simulink model "simulationInAccurateModel"  (R2022b)
settings: Solver=VariableStepAuto  StartTime=0.0  StopTime=20.0  MaxStep=2e-3  RelTol=1e-3
values from neighbouring files (symbols this model uses):
  K_c_PI1 = 0.15/k+(0.35-(theta*tau)/(theta+tau)^2)*(tau/(k*theta))    (= 1899030.33908)    [simulation.m]
  K_c_PI2 = 1/k*(tau/(tau/3+theta))    (= 2117647.05882)    [simulation.m]
  K_c_PID1 = 1/k*(0.2+0.45*(tau/theta))    (= 3440000)    [simulation.m]
  K_c_PID2 = 1/k*(2*tau+theta)/(2*tau/3+theta)    (= 2655172.41379)    [simulation.m]
  tau_d_PID1 = (0.5*theta*tau)/(0.3*theta+tau)    (= 0.12)    [simulation.m]
  tau_d_PID2 = (tau*theta)/(2*tau+theta)    (= 0.116883116883)    [simulation.m]
  tau_i_PI1 = 0.35*theta+(13*theta*tau^2)/(tau^2+12*theta*tau+7*theta^2)    (= 1.24751101625)    [simulation.m]
  tau_i_PI2 = tau    (= 1.8)    [simulation.m]
  tau_i_PID1 = theta*(0.4*theta+0.8*tau)/(theta+0.1*tau)    (= 0.895348837209)    [simulation.m]
  tau_i_PID2 = tau+theta/2    (= 1.925)    [simulation.m]
undefined symbols (not defined in the file or in its folder): k_over, k_under, tau_over, tau_under, theta_over, theta_under
settings Model: Creator=omare  LastModifiedBy=omare
settings DataIOCC: ReturnWorkspaceOutputs=off

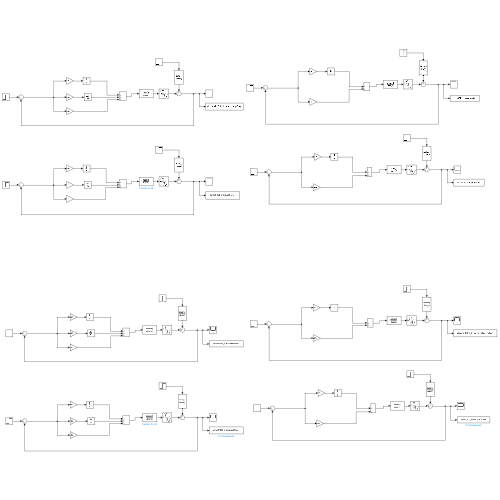
[thumbnail: Simulink's stored preview of the top-level diagram]
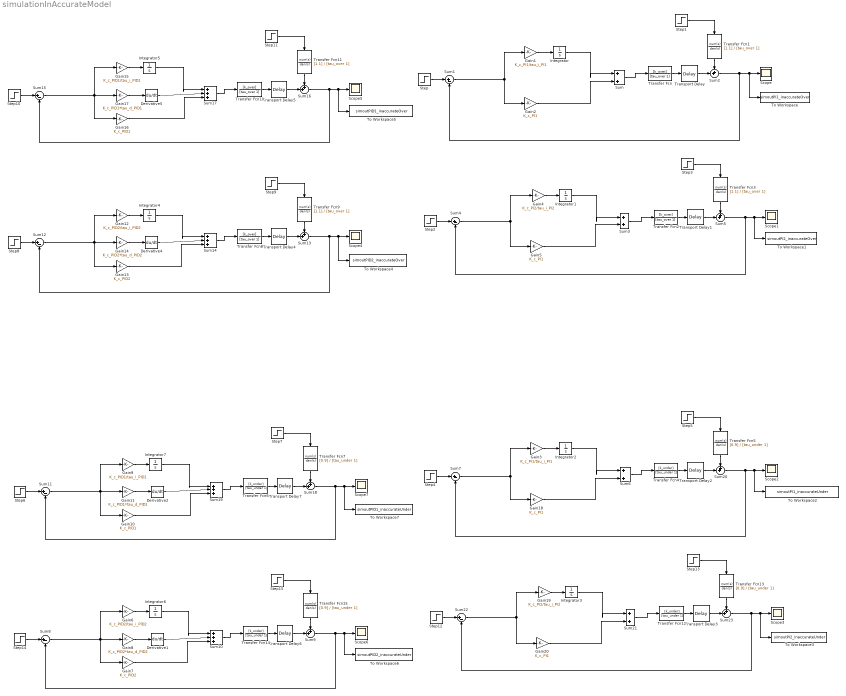
== system simulationInAccurateModel ==
  Derivative{1..2,4..5} (4 alike) : Derivative
  Gain1 : Gain  Gain=K_c_PI1/tau_i_PI1
  Gain10 : Gain  Gain=K_c_PID1
  Gain11 : Gain  Gain=K_c_PID1*tau_d_PID1
  Gain12 : Gain  Gain=K_c_PID2/tau_i_PID2
  Gain13 : Gain  Gain=K_c_PID2
  Gain14 : Gain  Gain=K_c_PID2*tau_d_PID2
  Gain15 : Gain  Gain=K_c_PID1/tau_i_PID1
  Gain16 : Gain  Gain=K_c_PID1
  Gain17 : Gain  Gain=K_c_PID1*tau_d_PID1
  Gain{2,5,18,20} (4 alike) : Gain  Gain=K_c_PI1
  Gain19 : Gain  Gain=K_c_PI2/tau_i_PI2
  Gain3 : Gain  Gain=K_c_PI1/tau_i_PI1
  Gain4 : Gain  Gain=K_c_PI2/tau_i_PI2
  Gain6 : Gain  Gain=K_c_PID2/tau_i_PID2
  Gain7 : Gain  Gain=K_c_PID2
  Gain8 : Gain  Gain=K_c_PID2*tau_d_PID2
  Gain9 : Gain  Gain=K_c_PID1/tau_i_PID1
  Integrator{,1..7} (8 alike) : Integrator
  Scope{,1..7} (8 alike) : Scope
  Step{,2,4,6,8,10,12,14} (8 alike) : Step  Time=0  SampleTime=0
  Step{1,3,5,7,9,11,13,15} (8 alike) : Step  Time=12  SampleTime=0
  Sum{,3,6,21} (4 alike) : Sum  Inputs=|++
  Sum{1,4,7..8,11..12,15,22} (8 alike) : Sum  Inputs=|+-
  Sum{10,14,17,19} (4 alike) : Sum  Inputs=|+++
  Sum{2,5,9,13,16,18,20,23} (8 alike) : Sum  Inputs=++|
  To Workspace : ToWorkspace  VariableName=simoutPI1_inaccurateOver  SaveFormat=Timeseries  SampleTime=-1
  To Workspace1 : ToWorkspace  VariableName=simoutPI2_inaccurateOver  SaveFormat=Timeseries  SampleTime=-1
  To Workspace2 : ToWorkspace  VariableName=simoutPI1_inaccurateUnder  SaveFormat=Timeseries  SampleTime=-1
  To Workspace3 : ToWorkspace  VariableName=simoutPI2_inaccurateUnder  SaveFormat=Timeseries  SampleTime=-1
  To Workspace4 : ToWorkspace  VariableName=simoutPID2_inaccurateOver  SaveFormat=Timeseries  SampleTime=-1
  To Workspace5 : ToWorkspace  VariableName=simoutPID1_inaccurateOver  SaveFormat=Timeseries  SampleTime=-1
  To Workspace6 : ToWorkspace  VariableName=simoutPID2_inaccurateUnder  SaveFormat=Timeseries  SampleTime=-1
  To Workspace7 : ToWorkspace  VariableName=simoutPID1_inaccurateUnder  SaveFormat=Timeseries  SampleTime=-1
  Transfer Fcn{,2,8,10} (4 alike) : TransferFcn  Numerator=[k_over]  Denominator=[tau_over 1]
  Transfer Fcn{1,3,9,11} (4 alike) : TransferFcn  Numerator=[1.1]  Denominator=[tau_over 1]
  Transfer Fcn{4,6,12,14} (4 alike) : TransferFcn  Numerator=[k_under]  Denominator=[tau_under 1]
  Transfer Fcn{5,7,13,15} (4 alike) : TransferFcn  Numerator=[0.9]  Denominator=[tau_under 1]
  Transport Delay{,1,4..5} (4 alike) : TransportDelay  DelayTime=theta_over
  Transport Delay{2..3,6..7} (4 alike) : TransportDelay  DelayTime=theta_under
  wires:
  Step2/1 -> Sum4/1
  Gain4/1 -> Integrator1/1
  Step/1 -> Sum1/1
  Integrator5/1 -> Sum17/1
  Derivative4/1 -> Sum14/2
  Transport Delay1/1 -> Sum5/2
  Sum16/1 -> To Workspace5/1, Scope5/1, Sum15/2
  Transfer Fcn10/1 -> Transport Delay5/1
  Transfer Fcn8/1 -> Transport Delay4/1
  Transport Delay4/1 -> Sum13/2
  Step8/1 -> Sum12/1
  Transfer Fcn9/1 -> Sum13/1
  Integrator/1 -> Sum/1
  Sum13/1 -> To Workspace4/1, Scope4/1, Sum12/2
  Integrator4/1 -> Sum14/1
  Sum15/1 -> Gain15/1, Gain16/1, Gain17/1
  Step10/1 -> Sum15/1
  Transfer Fcn11/1 -> Sum16/1
  Derivative5/1 -> Sum17/2
  Step11/1 -> Transfer Fcn11/1
  Gain15/1 -> Integrator5/1
  Gain16/1 -> Sum17/3
  Transport Delay5/1 -> Sum16/2
  Gain14/1 -> Derivative4/1
  Gain12/1 -> Integrator4/1
  Sum2/1 -> To Workspace/1, Scope/1, Sum1/2
  Sum17/1 -> Transfer Fcn10/1
  Sum/1 -> Transfer Fcn/1
  Transfer Fcn3/1 -> Sum5/1
  Transport Delay/1 -> Sum2/2
  Step3/1 -> Transfer Fcn3/1
  Gain17/1 -> Derivative5/1
  Sum1/1 -> Gain1/1, Gain2/1
  Sum3/1 -> Transfer Fcn2/1
  Step1/1 -> Transfer Fcn1/1
  Sum5/1 -> To Workspace1/1, Scope1/1, Sum4/2
  Transfer Fcn1/1 -> Sum2/1
  Sum4/1 -> Gain5/1, Gain4/1
  Gain13/1 -> Sum14/3
  Sum14/1 -> Transfer Fcn8/1
  Gain5/1 -> Sum3/2
  Transfer Fcn/1 -> Transport Delay/1
  Sum12/1 -> Gain12/1, Gain13/1, Gain14/1
  Gain1/1 -> Integrator/1
  Step9/1 -> Transfer Fcn9/1
  Integrator1/1 -> Sum3/1
  Transfer Fcn2/1 -> Transport Delay1/1
  Gain2/1 -> Sum/2
  Step12/1 -> Sum22/1
  Gain19/1 -> Integrator3/1
  Step4/1 -> Sum7/1
  Integrator7/1 -> Sum19/1
  Derivative1/1 -> Sum10/2
  Transport Delay3/1 -> Sum23/2
  Sum18/1 -> To Workspace7/1, Scope7/1, Sum11/2
  Transfer Fcn6/1 -> Transport Delay7/1
  Transfer Fcn14/1 -> Transport Delay6/1
  Transport Delay6/1 -> Sum9/2
  Step14/1 -> Sum8/1
  Transfer Fcn15/1 -> Sum9/1
  Integrator2/1 -> Sum6/1
  Sum9/1 -> To Workspace6/1, Scope6/1, Sum8/2
  Integrator6/1 -> Sum10/1
  Sum11/1 -> Gain9/1, Gain10/1, Gain11/1
  Step6/1 -> Sum11/1
  Transfer Fcn7/1 -> Sum18/1
  Derivative2/1 -> Sum19/2
  Step7/1 -> Transfer Fcn7/1
  Gain9/1 -> Integrator7/1
  Gain10/1 -> Sum19/3
  Transport Delay7/1 -> Sum18/2
  Gain8/1 -> Derivative1/1
  Gain6/1 -> Integrator6/1
  Sum20/1 -> To Workspace2/1, Scope2/1, Sum7/2
  Sum19/1 -> Transfer Fcn6/1
  Sum6/1 -> Transfer Fcn4/1
  Transfer Fcn13/1 -> Sum23/1
  Transport Delay2/1 -> Sum20/2
  Step13/1 -> Transfer Fcn13/1
  Gain11/1 -> Derivative2/1
  Sum7/1 -> Gain3/1, Gain18/1
  Sum21/1 -> Transfer Fcn12/1
  Step5/1 -> Transfer Fcn5/1
  Sum23/1 -> To Workspace3/1, Scope3/1, Sum22/2
  Transfer Fcn5/1 -> Sum20/1
  Sum22/1 -> Gain20/1, Gain19/1
  Gain7/1 -> Sum10/3
  Sum10/1 -> Transfer Fcn14/1
  Gain20/1 -> Sum21/2
  Transfer Fcn4/1 -> Transport Delay2/1
  Sum8/1 -> Gain6/1, Gain7/1, Gain8/1
  Gain3/1 -> Integrator2/1
  Step15/1 -> Transfer Fcn15/1
  Integrator3/1 -> Sum21/1
  Transfer Fcn12/1 -> Transport Delay3/1
  Gain18/1 -> Sum6/2
